simulink model "aCLF_ClosedLoop"  (R2024b)
settings: Solver=ode45  StartTime=0.0  StopTime=60  RelTol=1e-6  AbsTol=1e-8
settings Model: Creator=LAPTOPASADI  LastModifiedBy=LAPTOPASADI

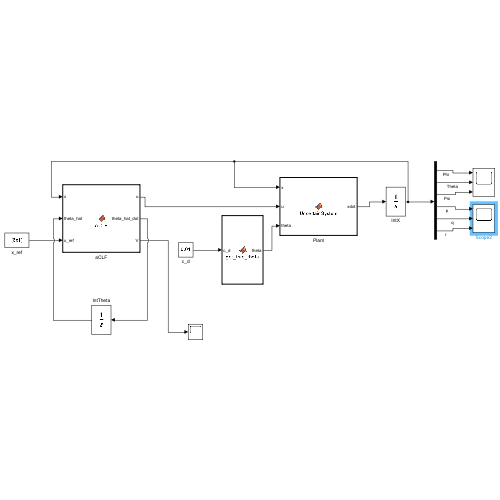
[thumbnail: Simulink's stored preview of the top-level diagram]
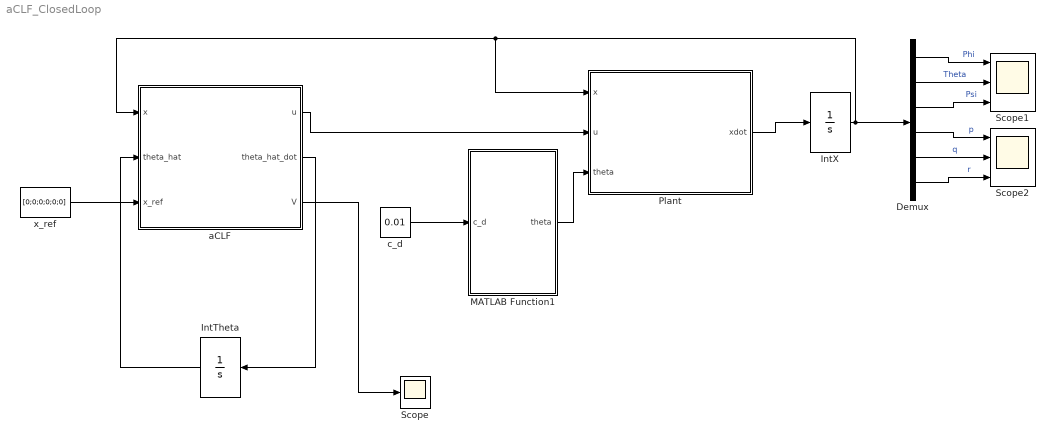
== system aCLF_ClosedLoop ==
  Demux : Demux  Outputs=6
  IntTheta : Integrator  InitialCondition=[0;0.5;0.5;0;-0.3;0]
  IntX : Integrator  InitialCondition=[deg2rad(10);0;deg2rad(30);0.5;0.4;0]
  MATLAB Function1 : MATLAB Function  TreatAsAtomicUnit=on
  Plant : MATLAB Function  TreatAsAtomicUnit=on
  Scope : Scope
  Scope1 : Scope  NumInputPorts=3
  Scope2 : Scope  NumInputPorts=3
  aCLF : MATLAB Function  TreatAsAtomicUnit=on
  c_d : Constant  Value=0.01
  x_ref : Constant  Value=[0;0;0;0;0;0]
  wires:
  IntX/1 -> Demux/1, aCLF/1(x), Plant/1(x)
  IntTheta/1 -> aCLF/2(theta_hat)
  x_ref/1 -> aCLF/3(x_ref)
  aCLF/1(u) -> Plant/2(u)
  aCLF/2(theta_hat_dot) -> IntTheta/1
  Plant/1(xdot) -> IntX/1
  aCLF/3(V) -> Scope/1
  c_d/1 -> MATLAB Function1/1(c_d)
  MATLAB Function1/1(theta) -> Plant/3(theta)
  Demux/4 -> Scope2/1  "p"
  Demux/6 -> Scope2/3  "r"
  Demux/2 -> Scope1/2  "Theta"
  Demux/5 -> Scope2/2  "q"
  Demux/1 -> Scope1/1  "Phi"
  Demux/3 -> Scope1/3  "Psi"

== matlab function aCLF_ClosedLoop/aCLF ==
  data: x input; u output; theta_hat input; x_ref input; theta_hat_dot output; V output
function [u, theta_hat_dot, V] = aCLF(x, theta_hat, x_ref)
%#codegen
    coder.extrinsic('lyap','quadprog','optimoptions');

    gamma_clf = 0.5;
    Gamma     = 10*eye(6);
    u_min     = -0.1;  u_max = 0.1;

    Ixx = 0.0043;  Iyy = 0.0142;  Izz = 0.0176;  Ixz = 1e-4;
    dcg = 0.175;   hcg = 0.085;   d_over_b = 1.2e-6/3.13e-5;
    I = [ Ixx,0,-Ixz; 0,Iyy,0; -Ixz,0,Izz];
    B_alloc = [0,0,dcg,d_over_b;  0,hcg,0,0;  0,0,d_over_b,-dcg];
    Acl = [zeros(3),eye(3); -4*eye(3),-4*eye(3)];
    P = zeros(6);  P = lyap(Acl', 0.1*eye(6));

    phi = x(1);  th = x(2);
    p = x(4);  q = x(5);  r = x(6);
    omega = [p; q; r];

    y = [phi; th; x(3)] - x_ref(1:3);
    [J, dJdphi, dJdth] = euler_J(phi, th);
    y_dot = J*omega;

    eta = [y; y_dot];
    V   = eta'*P*eta;
    P11 = P(1:3,1:3); P12 = P(1:3,4:6); P22 = P(4:6,4:6);

    J_dot  = dJdphi*y_dot(1) + dJdth*y_dot(2);
    alpha0 = J_dot*omega;

    F_omega = [ p*q,-q*r,0,0,0,-p;  0,0,p*r,-(p^2-r^2),0,-q;  -q*r,0,0,0,p*q,-r];
    G_omega = I \ B_alloc;
    alpha_F = J * F_omega;
    A_dec   = J * G_omega;

    sigma     = 2*(y'*P12 + y_dot'*P22);
    omega_clf = 2*(y'*P11 + y_dot'*P12')*y_dot + sigma*alpha0;
    phi_clf   = alpha_F' * sigma';
    LgV       = sigma * A_dec;

    b_clf = -omega_clf - phi_clf'*theta_hat - gamma_clf*V;

    H    = 2*eye(4);
    f_qp = zeros(4,1);
    lb   = u_min*ones(4,1);
    ub   = u_max*ones(4,1);
    opts = optimoptions('quadprog','Display','off');

    u    = zeros(4,1);
    flag = 0;
    [u, ~, flag] = quadprog(H, f_qp, LgV, b_clf, [], [], lb, ub, [], opts);
    if flag < 0, u = zeros(4,1); end

    theta_hat_dot = Gamma * phi_clf;
end

function [J, dJdphi, dJdth] = euler_J(phi, th)
    cphi = cos(phi);  sphi = sin(phi);
    cth  = cos(th);   sth  = sin(th);
    if abs(cth) < 1e-6, cth = sign(cth + 1e-6)*1e-6; end
    tth = sth/cth;  sec2 = 1/cth^2;
    J      = [1, sphi*tth, cphi*tth;  0, cphi, -sphi;  0, sphi/cth, cphi/cth];
    dJdphi = [0, cphi*tth,-sphi*tth;  0,-sphi,-cphi;   0, cphi/cth,-sphi/cth];
    dJdth  = [0, sphi*sec2,    cphi*sec2;
              0, 0,            0;
              0, sphi*sth*sec2,cphi*sth*sec2];
end

== matlab function aCLF_ClosedLoop/Plant ==
  data: x input; u input; xdot output; theta input
function xdot = UncertainSystem(x, u, theta)
%#codegen
% MATLAB Function block for  Uncertain_System.slx.
% Inputs : x (6), u (4), theta (6)
% Output : xdot (6) so that  xdot = f0(x) + F(x)*theta + g(x)*u.

    Ixx = 0.0043;  Iyy = 0.0142;  Izz = 0.0176;  Ixz = 1e-4;
    dcg = 0.175;   hcg = 0.085;   d_over_b = 1.2e-6 / 3.13e-5;

    I = [ Ixx, 0, -Ixz;  0, Iyy, 0;  -Ixz, 0, Izz];
    B_alloc = [0, 0,   dcg,        d_over_b;
               0, hcg, 0,          0;
               0, 0,   d_over_b,  -dcg];

    phi = x(1);  th = x(2);
    p   = x(4);  q  = x(5);  r = x(6);
    omega = [p; q; r];

    cphi = cos(phi);  sphi = sin(phi);
    cth  = cos(th);   sth  = sin(th);
    if abs(cth) < 1e-6, cth = sign(cth + 1e-6)*1e-6; end
    tth = sth/cth;

    J = [1, sphi*tth, cphi*tth;
         0, cphi,    -sphi;
         0, sphi/cth, cphi/cth];

    F_omega = [ p*q, -q*r, 0,    0,           0,   -p;
                0,    0,   p*r, -(p^2 - r^2), 0,   -q;
               -q*r,  0,   0,    0,           p*q, -r];

    f0    = [J*omega; 0; 0; 0];
    F_reg = [zeros(3,6); F_omega];
    g     = [zeros(3,4); I \ B_alloc];

    xdot = f0 + F_reg*theta + g*u;
end

== matlab function aCLF_ClosedLoop/MATLAB Function1 ==
  data: c_d input; theta output
function theta = get_true_theta(c_d)
    
    Ixx = 0.0043;
    Iyy = 0.0142;
    Izz = 0.0176;
    Ixz = 0.0001;

    Gam = Ixx * Izz - Ixz^2;

    Gam1 = (Ixz * (Ixx - Iyy + Izz)) / Gam;
    Gam2 = (Izz * (Izz - Iyy) + Ixz^2) / Gam;
    Gam5 = (Izz - Ixx) / Iyy;
    Gam6 = Ixz / Iyy;
    Gam7 = ((Ixx - Iyy) * Ixx + Ixz^2) / Gam;

    theta = [Gam1; Gam2; Gam5; Gam6; Gam7; c_d];

end
